simulink model "gradMRAC_1rad_R2016a"  (R2016a)
settings: Solver=ode45  StartTime=0.0  StopTime=100  FixedStep=SIMstepSize  RelTol=1e-3
values from neighbouring files (symbols this model uses):
  a0 = 0.55    [gradMRAC_1rad_PARAMETRE.m]
  a0m = 1    [gradMRAC_1rad_PARAMETRE.m]
  b0m = 1    [gradMRAC_1rad_PARAMETRE.m]
settings Model: Creator=MT  LastModifiedBy=MT
settings DataIOCC: LimitDataPoints=on  SaveFormat=Array  SignalLoggingSaveFormat=ModelDataLogs  SaveOutput=off  SignalLogging=off  DSMLogging=off  SaveTime=off
settings OptimizationCC: ExpressionDepthLimit=2147483647
settings DebuggingCC: UnderspecifiedInitializationDetection=Classic  MergeDetectMultiDrivingBlocksExec=none  SolverPrmCheckMsg=warning  FcnCallInpInsideContextMsg=EnableAllAsWarning  StateNameClashWarn=warning
settings HardwareCC: ProdBitPerPointer=32  ProdLargestAtomicFloat=None  ProdIntDivRoundTo=Undefined  ProdEndianess=Unspecified  ProdWordSize=32  ProdHWDeviceType=32-bit Generic
settings ModelReferenceCC: PropagateSignalLabelsOutOfModel=off
settings GRTTargetCC: CombineOutputUpdateFcns=off  GRTInterface=on

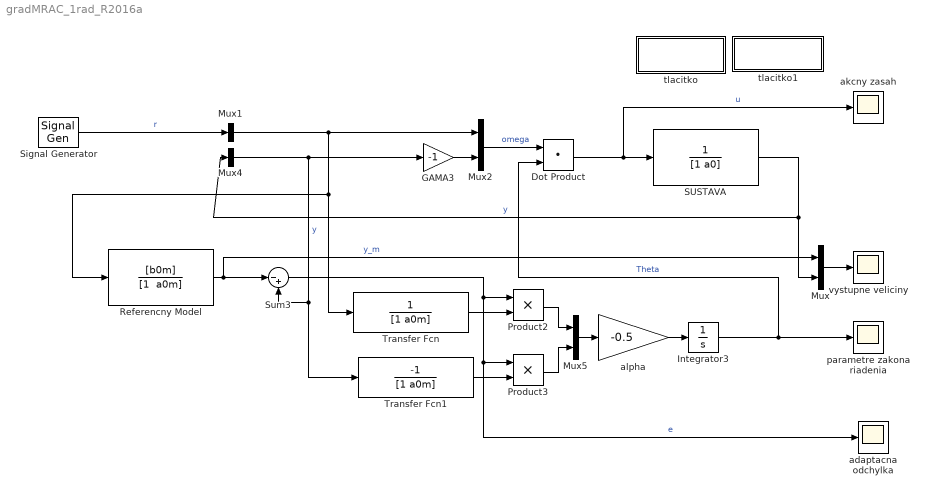
== system gradMRAC_1rad_R2016a ==
  Dot Product : DotProduct  InputSameDT=on  OutDataTypeStr=Inherit: Inherit via internal rule
  GAMA3 : Gain  Gain=-1
  Integrator3 : Integrator
  Mux : Mux  Inputs=2
  Mux1 : Mux  Inputs=1
  Mux2 : Mux  Inputs=2
  Mux4 : Mux  Inputs=1
  Mux5 : Mux  Inputs=2
  Product2 : Product  RndMeth=Zero
  Product3 : Product  RndMeth=Zero
  Referencny Model : TransferFcn  Numerator=[b0m]  Denominator="[1  a0m]"
  SUSTAVA : TransferFcn  Denominator=[1 a0]
  Signal Generator : SignalGenerator  WaveForm=square  Amplitude=-1  Frequency=0.05
  Sum3 : Sum  Inputs=|-+
  Transfer Fcn : TransferFcn  Denominator=[1 a0m]
  Transfer Fcn1 : TransferFcn  Numerator=[-1]  Denominator=[1 a0m]
  adaptacna odchylka : Scope
  akcny zasah : Scope
  alpha : Gain  Gain=-0.5
  parametre zakona riadenia : Scope
  tlacitko : Subsystem
      settings: OpenFcn=gradMRAC_1rad_PARAMETRE
      mask Display: fprintf('nacitat\nPARAMETRE')
  tlacitko1 : Subsystem
      settings: OpenFcn=open gradMRAC_1rad_PARAMETRE.m
      mask Display: fprintf('zmenit\nPARAMETRE')
  vystupne veliciny : Scope
  wires:
  Mux/1 -> vystupne veliciny/1
  Signal Generator/1 -> Mux1/1  "r"
  Referencny Model/1 -> Sum3/1, Mux/1  "y_m"
  Mux1/1 -> Mux2/1, Transfer Fcn/1, Referencny Model/1
  Product2/1 -> Mux5/1
  Product3/1 -> Mux5/2
  SUSTAVA/1 -> Mux/2, Mux4/1  "y"
  Mux2/1 -> Dot Product/1  "omega"
  Mux4/1 -> Transfer Fcn1/1, Sum3/2, GAMA3/1  "y"
  Transfer Fcn/1 -> Product2/2
  Transfer Fcn1/1 -> Product3/2
  Sum3/1 -> Product2/1, Product3/1, adaptacna odchylka/1  "e"
  Dot Product/1 -> SUSTAVA/1, akcny zasah/1  "u"
  GAMA3/1 -> Mux2/2
  Mux5/1 -> alpha/1
  Integrator3/1 -> parametre zakona riadenia/1, Dot Product/2  "Theta"
  alpha/1 -> Integrator3/1

== system gradMRAC_1rad_R2016a/tlacitko ==

== system gradMRAC_1rad_R2016a/tlacitko1 ==
